simulink model "xmc_video_frame_rotation"  (R2023a)
settings: Solver=VariableStepAuto  StartTime=0.0  StopTime=inf  RelTol=1e-3  EnableMultiTasking=on
PostLoadFcn:
  | xmcHubUpdateInstalledDevice(gcs);
undefined symbols (not defined in the file): A, AXI4, N, Stream, xc7vx485tffg1157
libraries: visionsinks x3, vmcUtilities x2, video_frame_rotation_lib x2, dspvision x1, hlsUtilities x1
settings Model: Creator=dvancamp  LastModifiedBy=robg
settings SolverCC: AlgebraicLoopSolver=TrustRegion
settings DataIOCC: LimitDataPoints=on  ReturnWorkspaceOutputs=off
settings OptimizationCC: LifeSpan=inf
settings DebuggingCC: UnconnectedInputMsg=warning  UnconnectedOutputMsg=warning  UnconnectedLineMsg=warning  AllowSymbolicDim=off  SFUnexpectedBacktrackingDiag=warning  SFNoUnconditionalDefaultTransitionDiag=warning  SFExecutionAtInitializationDiag=none  ArithmeticOperatorsInVariantConditions=warning
settings ModelReferenceCC: EnableRefExpFcnMdlSchedulingChecks=on  PropagateSignalLabelsOutOfModel=off
settings SFSimCC: SimUseLocalCustomCode=off  CustomCodeUndefinedFunction=UseInterfaceOnly
settings RTWCC: RTWUseLocalCustomCode=off  DLArmComputeVersion=19.05
settings CodeAppCC: StateflowObjectComments=on
settings GRTTargetCC: TargetLangStandard=C89/C90 (ANSI)
settings ConfigComp: CovMetricSettings=dw  CovSaveCumulativeToWorkspaceVar=on  CovSaveSingleToWorkspaceVar=on  CovExternalEMLEnable=off

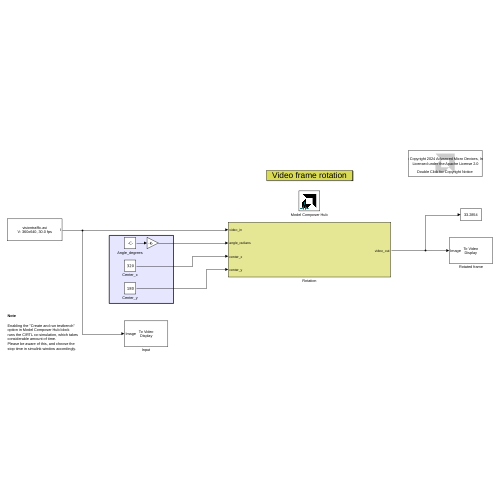
[thumbnail: Simulink's stored preview of the top-level diagram]
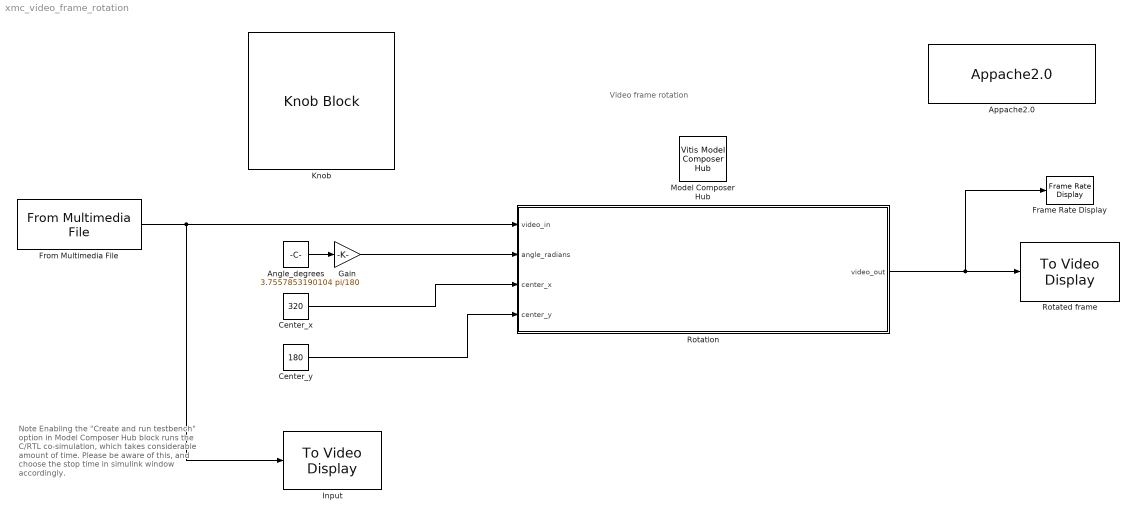
== system xmc_video_frame_rotation ==
  note: Note
      |
      | Enabling the "Create and run testbench" option in Model Composer Hub block
      | runs the C/RTL co-simulation, which takes considerable amount of time.
      | Please be aware of this, and choose the stop time in simulink window accordingly.
  note: Video frame rotation
  Angle_degrees : Constant  Value=3.7557853190104  OutDataTypeStr=single  SampleTime=-1
  Appache2.0 : vmcUtilities/Appache2.0
  Center_x : Constant  Value=320  OutDataTypeStr=single  SampleTime=-1
  Center_y : Constant  Value=180  OutDataTypeStr=single  SampleTime=-1
  Frame Rate Display : visionsinks/Frame Rate Display  UpdateRate=10
  From Multimedia File : dspvision/From Multimedia File  inputFilename=visiontraffic.avi  readRange=[1 Inf]  loop=on  numPlays=inf  outputStreams=Video only  videoDataType=uint8  audioDataType=int16  inheritSampleTime=off  userDefinedSampleTime=1/30  noAudioOutput=off  isIntensityVideo=off  fourcc=Intensity  colorVideoFormat=One multidimensional signal  outputEOF=off  dataOrg=Column-major  audioFrameSize=1024  computeAudioFrameSize=off  outSamplingMode=Sample based
  Gain : Gain  Gain=pi/180
  Input : visionsinks/To Video Display  windowSizeMode=Normal  openAtMdlStart=on  fullScreen=off  videoWindowX=141  videoWindowY=382  saveWindowSize=off  videoWindowWidth=613  videoWindowHeight=348  inputColorFormat=RGB  inputType=Obsolete  imagePorts=One multidimensional signal  OutputDevice=On-screen video monitor  dataOrg=Column-major  isWindowOpen=off
  Knob : KnobBlock  ScaleMax=8  TickInterval=1
  Model Composer Hub : vmcUtilities/Vitis Model Composer Hub  Tag=genX  CodeGeneration=off  SubsystemName=Rotation  StartColumn=1  NumberOfColumns=1  TargetDirectory=./code  exportDesign=off  analyzeDesign=off  validateDesignOnHw=off  ExportType=IP Catalog  IpVendor=xilinx.com  IpLibrary=hls  IpVersion=1.0  IpHWLanguage=Verilog  AieCompilerOptions={}  AieSimulatorOptions={}  CreateTestbench=off  TestbenchStackSize=10  RunRtlSim=off  RunCSim=off  RunAieSim=off  AieSimTimeout=50000  RunAieSimProfiling=off  LaunchVitisAnalyzer=off  PlotOutput=off  RunX86Sim=on  X86SimTimeout=10  GenHwImage=off  GenLibadfXo=off  GenHwValidationCode=off  PlatformType=Not Specified  HwSystemType=Baremetal  HwValidationTarget=hw  ProjDevice=xc7vx485tffg1157-1  ProjDevicePart=xc7vx485tffg1157-1  SamplePeriod=-1  ClockFrequency=200  DataPathParallelism=1  xilinxfamily=Kintex7  part=xc7k325t  speed=-3  package=fbg676  directory=./netlist  testbench=off  incr_netlist=off  synthesis_tool=Vivado  clock_wrapper=Clock Enables  dbl_ovrd=According to Block Masks  dcm_input_clock_period=10  sysclk_period=10  simulink_period=1  eval_field=0  LogFileName=''  NThreads=4
  Rotated frame : visionsinks/To Video Display  windowSizeMode=True size (1:1)  openAtMdlStart=on  fullScreen=off  videoWindowX=861  videoWindowY=370  saveWindowSize=off  videoWindowWidth=640  videoWindowHeight=360  inputColorFormat=RGB  inputType=Obsolete  imagePorts=One multidimensional signal  OutputDevice=On-screen video monitor  dataOrg=Column-major  isWindowOpen=off
  Rotation : Subsystem
  wires:
  From Multimedia File/1 -> Input/1, Rotation/1(video_in)
  Rotation/1(video_out) -> Frame Rate Display/1, Rotated frame/1
  Angle_degrees/1 -> Gain/1
  Gain/1 -> Rotation/2(angle_radians)
  Center_x/1 -> Rotation/3(center_x)
  Center_y/1 -> Rotation/4(center_y)

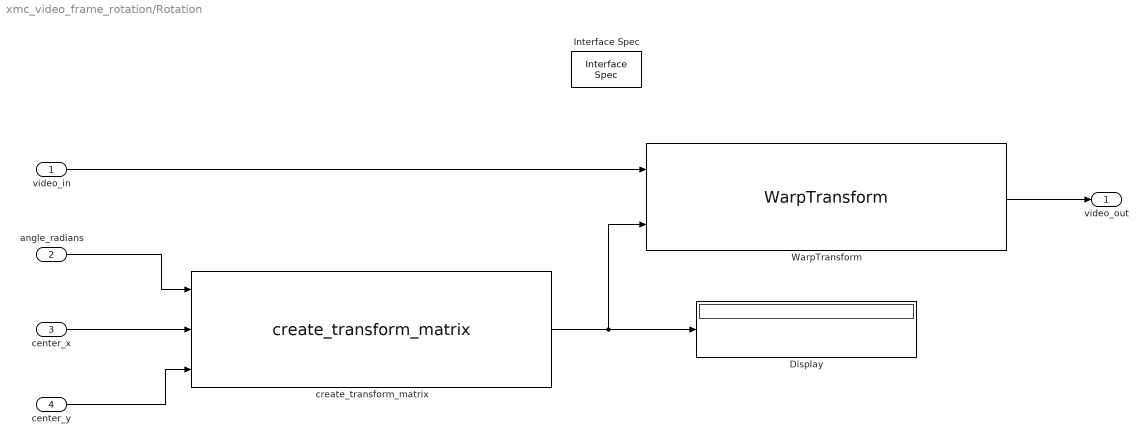
== system xmc_video_frame_rotation/Rotation ==
  video_in : Inport
  angle_radians : Inport  Port=2
  center_x : Inport  Port=3
  center_y : Inport  Port=4
  Display : Display
  Interface Spec : hlsUtilities/Interface Spec  Return=AXI4-Lite Slave@rotation_ctrl@  InportInterfaces={'AXI4-Stream@@@N/A@N/A', 'AXI4-Lite Slave@rotation_ctrl@@N/A@N/A', 'AXI4-Lite Slave@rotation_ctrl@@N/A@N/A', 'AXI4-Lite Slave@rotation_ctrl@@N/A@N/A'}  InportHandles={4.706012695312500000e+03, 4.708013061523437500e+03, 4.710014160156250000e+03, 4.712013427734375000e+03}  InportNames={'video_in', 'angle_radians', 'center_x', 'center_y'}  OutportInterfaces={'AXI4-Stream@@@N/A@N/A'}  OutportHandles={4.726013549804687500e+03}  OutportNames={'video_out'}  Mode=AXI4-Lite Slave  Bundle=rotation_ctrl  InName1=video_in  InMode1=AXI4-Stream  InVFormat1=N/A  InVComponent1=N/A  InName2=angle_radians  InMode2=AXI4-Lite Slave  InBundle2=rotation_ctrl  InVFormat2=N/A  InVComponent2=N/A  InName3=center_x  InMode3=AXI4-Lite Slave  InBundle3=rotation_ctrl  InVFormat3=N/A  InVComponent3=N/A  InName4=center_y  InMode4=AXI4-Lite Slave  InBundle4=rotation_ctrl  InVFormat4=N/A  InVComponent4=N/A  InName5=center_y  InMode5=AXI4-Lite Slave  InBundle5=rotation_control  InVFormat5=N/A  InVComponent5=N/A  InMode6=Default  InVFormat6=N/A  InVComponent6=N/A  InMode7=Default  InVFormat7=N/A  InVComponent7=N/A  InMode8=Default  InVFormat8=N/A  InVComponent8=N/A  OutName1=video_out  OutMode1=AXI4-Stream  OutVFormat1=N/A  OutVComponent1=N/A  OutMode2=Default  OutVFormat2=N/A  OutVComponent2=N/A  OutMode3=Default  OutVFormat3=N/A  OutVComponent3=N/A  OutMode4=Default  OutVFormat4=N/A  OutVComponent4=N/A  OutMode5=Default  OutVFormat5=N/A  OutVComponent5=N/A  OutMode6=Default  OutVFormat6=N/A  OutVComponent6=N/A  OutMode7=Default  OutVFormat7=N/A  OutVComponent7=N/A  OutMode8=Default  OutVFormat8=N/A  OutVComponent8=N/A
  WarpTransform : video_frame_rotation_lib/WarpTransform  LibraryFunction=WarpTransform  IncludeFiles={'warp_transform_wrap.h'}  SourceFiles={}  IncludeDirectories={'./include'}  TemplateParams={'int ROWS'; 'int COLS'; 'int NPC'}  FunctionParamTypes={xmcDataType('void'); xmcDataType('uint8_t'); xmcDataType('float'); xmcDataType('uint8_t'); xmcDataType('int')}  FunctionParamPassbys={0.000000000000000000e+00; 0.000000000000000000e+00; 0.000000000000000000e+00; 0.000000000000000000e+00; 0.000000000000000000e+00}  FunctionParamDimensions={'1'; '[ROWS][COLS]'; '[9]'; '[ROWS][COLS]'; '1'}  FunctionParamNames={'return'; 'video_in'; 'T_matrix'; 'video_out'; 'NPC'}  FunctionParamDir={0.000000000000000000e+00; 1.000000000000000000e+00; 1.000000000000000000e+00; 2.000000000000000000e+00; 3.000000000000000000e+00}  FunctionParamSupportsStreaming={true; true; true; true; true}  BufferDepth={'0'}  FunctionParamValues={'0'; '0'; '0'; '0'; '0'}  ThroughputFactors={''}  NPC=1
  create_transform_matrix : video_frame_rotation_lib/create_transform_matrix  LibraryFunction=create_transform_matrix  IncludeFiles={'create_transform_matrix.h'}  SourceFiles={}  IncludeDirectories={}  TemplateParams={' '}  FunctionParamTypes={xmcDataType('void'); xmcDataType('const float'); xmcDataType('const float'); xmcDataType('const float'); xmcDataType('float')}  FunctionParamPassbys={0.000000000000000000e+00; 0.000000000000000000e+00; 0.000000000000000000e+00; 0.000000000000000000e+00; 0.000000000000000000e+00}  FunctionParamDimensions={'1'; '1'; '1'; '1'; '[9]'}  FunctionParamNames={'return'; 'angle'; 'center_x'; 'center_y'; 'transform_matrix'}  FunctionParamDir={0.000000000000000000e+00; 1.000000000000000000e+00; 1.000000000000000000e+00; 1.000000000000000000e+00; 2.000000000000000000e+00}  FunctionParamSupportsStreaming={true; true; true; true; true}  BufferDepth={'0'}  FunctionParamValues={'0'; '0'; '0'; '0'; '0'}  ThroughputFactors={''}
  video_out : Outport  VectorParamsAs1DForOutWhenUnconnected=off
  wires:
  video_in/1 -> WarpTransform/1
  WarpTransform/1 -> video_out/1
  create_transform_matrix/1 -> Display/1, WarpTransform/2
  angle_radians/1 -> create_transform_matrix/1
  center_x/1 -> create_transform_matrix/2
  center_y/1 -> create_transform_matrix/3
